simulink model "Vehicle_model_testing"  (R2016b)
settings: Solver=ode3  StartTime=0.0  StopTime=50  RelTol=1e-3
settings Model: Creator=liana  LastModifiedBy=liana

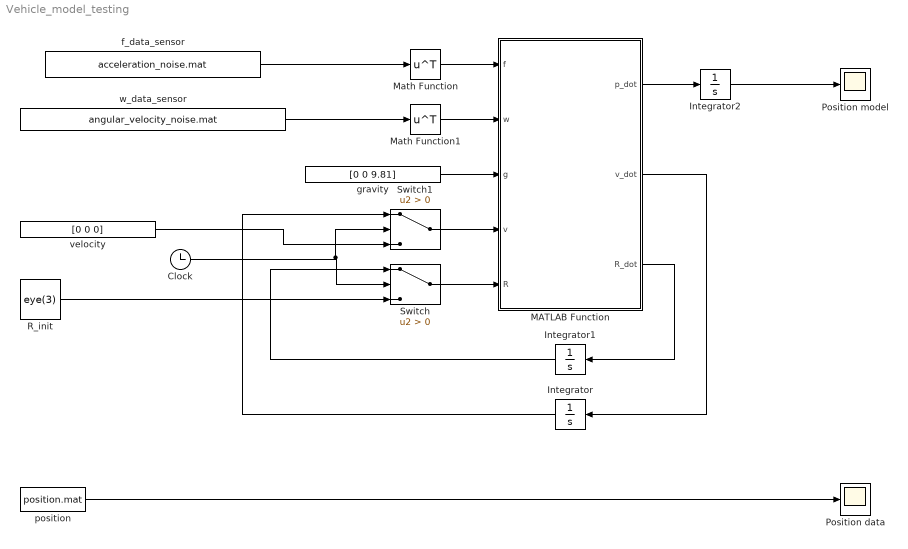
== system Vehicle_model_testing ==
  Clock : Clock
  Integrator : Integrator
  Integrator1 : Integrator
  Integrator2 : Integrator
  MATLAB Function : MATLAB Function  TreatAsAtomicUnit=on
  Math Function : Math  Operator=transpose  SaturateOnIntegerOverflow=on
  Math Function1 : Math  Operator=transpose  SaturateOnIntegerOverflow=on
  Position data : Scope
  Position model : Scope
  R_init : Constant  Value=eye(3)  VectorParams1D=off  SampleTime=-1
  Switch : Switch  Criteria=u2 > Threshold
  Switch1 : Switch  Criteria=u2 > Threshold
  f_data_sensor : FromFile  FileName=acceleration_noise.mat  SampleTime=0
  gravity : Constant  Value=[0 0 9.81]
  position : FromFile  FileName=position.mat  SampleTime=0
  velocity : Constant  Value=[0 0 0]
  w_data_sensor : FromFile  FileName=angular_velocity_noise.mat  SampleTime=0
  wires:
  w_data_sensor/1 -> Math Function1/1
  f_data_sensor/1 -> Math Function/1
  MATLAB Function/3(R_dot) -> Integrator1/1
  MATLAB Function/2(v_dot) -> Integrator/1
  MATLAB Function/1(p_dot) -> Integrator2/1
  Integrator2/1 -> Position model/1
  Math Function/1 -> MATLAB Function/1(f)
  Math Function1/1 -> MATLAB Function/2(w)
  gravity/1 -> MATLAB Function/3(g)
  Clock/1 -> Switch1/2, Switch/2
  R_init/1 -> Switch/3
  Integrator1/1 -> Switch/1
  Switch/1 -> MATLAB Function/5(R)
  Integrator/1 -> Switch1/1
  Switch1/1 -> MATLAB Function/4(v)
  velocity/1 -> Switch1/3
  position/1 -> Position data/1

== matlab function Vehicle_model_testing/MATLAB Function ==
  data: f input size=[3,1]; w input size=[3,1]; g input size=[3,1]; v input size=[3,1]; p_dot output size=[3,1]; R input size=[3,3]; v_dot output size=[3,1]; R_dot output size=[3,3]
function [p_dot, v_dot, R_dot] = Vehicle_Model(f,w,g,v,R)

    p_dot = v;
    v_dot = R*f+g;
    R_dot = R*skew(w);

;
